simulink model "lab_3"  (R2015a)
settings: Solver=ode45  StartTime=0.0  StopTime=inf  RelTol=1e-3
InitFcn:
  | clc;
  | close all;
  | clear all;
  | 
  | Ts = 1;
  | Nc = 10000;
  | 
  | Nstart = 10;
  | Nend = 20;
  | 
  | Range = [Nstart Nend];
  | qs=[1/6 2/5 2/3];
  | 
  | time_vals = zeros(1, Nc);
  | char_vals = zeros(1,Nc);
  | 
  | pause_t=0.3;
StartFcn:
  | disp('Opening the RS232 port . . . . . ');
  | 
  | s_port = serial('COM4', 'BaudRate', 9600, 'Parity', 'none');
  | set(s_port, 'InputBufferSize', 1);
  | set(s_port, 'OutputBufferSize', 1);
  | fopen(s_port);
  | 
  | disp('RS232 port activated!');
StopFcn:
  | disp('Closing the RS232 port . . . . . ');
  | 
  | fclose(s_port);
  | delete(s_port);
  | clear s_port;
  | 
  | disp('RS232 port closed!');
  | 
  | %for i = 1:Nc-1
  |   %diff(i) = time_vals(i+1) - time_vals(i);
  | %end
  | 
  | %x = 1:7;
  | 
  | %hist(diff,x)
settings Model: Creator=ees1504  LastModifiedBy=tamias
settings OptimizationCC: ExpressionDepthLimit=2147483647
settings DebuggingCC: UnderspecifiedInitializationDetection=Classic  MergeDetectMultiDrivingBlocksExec=none  SolverPrmCheckMsg=warning  StateNameClashWarn=warning
settings GRTTargetCC: CombineOutputUpdateFcns=off  GRTInterface=on

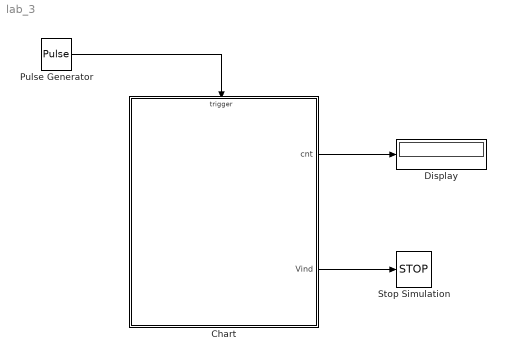
== system lab_3 ==
  Chart : Stateflow chart  TreatAsAtomicUnit=on
  Display : Display
  Pulse Generator : DiscretePulseGenerator  PulseType=Time based  Period=Ts  PulseWidth=50
  Stop Simulation : Stop
  wires:
  Chart/1(cnt) -> Display/1
  Chart/2(Vind) -> Stop Simulation/1
  Pulse Generator/1 -> Chart/Trigger

== stateflow chart lab_3/Chart ==
  state C [parallel]
    settings: executionOrder=1
    state UpCounter
      entry: upc = upc + 1;
      during: upc = upc + 1;
      UpCounter -> UpCounter
    (default) -> UpCounter : {upc=0;}
  state D [parallel]
    settings: executionOrder=2
    state S0
      entry: cnt = cnt + 1;
      ml.char_vals[cnt] = ml.randi(ml.Range, 1, 1);
      ml.fwrite(ml.s_port, ml.char_vals[cnt], 'uchar');
      ml.time_vals[cnt] = upc;
      ml.pause(ml.pause_t);
    state S_end
      entry: Vind = 1;
    state S1
      ml.pause(ml.pause_t);
    state S4
      ml.pause(ml.pause_t);
    state S3
      ml.pause(ml.pause_t);
    state S5
      ml.pause(ml.pause_t);
    state S2
      ml.pause(ml.pause_t);
    (default) -> S0 : {cnt=0;Vind=0;}
    S0 -> S_end [order 1] : [cnt==ml.Nc]
    (junction 70) -> S0
    S0 -> S1 [order 2]
    S3 -> S4
    S1 -> (junction 28) : {val=ml.rand(1);}
    S4 -> (junction 61) : {val=ml.rand(1);}
    S5 -> (junction 70)
    (junction 61) -> S5 [order 1] : [val>ml.qs[3]]
    (junction 34) -> S3 [order 1] : [val>ml.qs[2]]
    (junction 28) -> S2 [order 2] : [val>ml.qs[1]]
    S2 -> (junction 34) : {val=ml.rand(1);}
    (junction 34) -> (junction 70) [order 2] : [val<=ml.qs[2]]
    (junction 28) -> (junction 70) [order 1] : [val<=ml.qs[1]]
    (junction 61) -> (junction 70) [order 2] : [val<=ml.qs[3]]
  data: val local double; cnt output double; Vind output boolean; upc local int32
  events: clk input RISING_EDGE_EVENT
